simulink model "PI"  (R2020b)
settings: Solver=VariableStepAuto  StartTime=0.0  StopTime=10  RelTol=1e-3
values from neighbouring files (symbols this model uses):
  Ki = 40    [w2_prob2matfile.m]
  Kp = 800    [w2_prob2matfile.m]
  Ts = 0.01    [w2_prob2matfile.m]
settings Model: Creator=Akshay A H  LastModifiedBy=Akshay A H
settings DataIOCC: SaveOutput=off  SaveTime=off

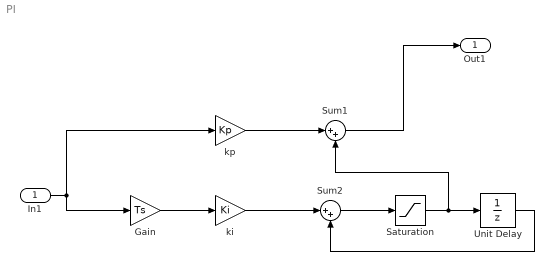
== system PI ==
  In1 : Inport  OutDataTypeStr=double  PortDimensions=1  SampleTime=0
  Gain : Gain  Gain=Ts
  Saturation : Saturate  UpperLimit=1  LowerLimit=1
  Sum1 : Sum  Inputs=|++
  Sum2 : Sum  Inputs=|++
  Unit Delay : UnitDelay  SampleTime=-1  HasFrameUpgradeWarning=on
  ki : Gain  Gain=Ki
  kp : Gain  Gain=Kp
  Out1 : Outport  OutDataTypeStr=double  PortDimensions=1  SampleTime=0
  wires:
  ki/1 -> Sum2/1
  Unit Delay/1 -> Sum2/2
  Sum2/1 -> Saturation/1
  In1/1 -> kp/1, Gain/1
  Saturation/1 -> Unit Delay/1, Sum1/2
  Gain/1 -> ki/1
  kp/1 -> Sum1/1
  Sum1/1 -> Out1/1
